simulink model "Tractor_BURGERS_etrailer_v2_1_backup070824"  (R2023a)
settings: Solver=VariableStepAuto  StartTime=0.0  StopTime=tmax  FixedStep=dt  RelTol=1e-3  EnableMultiTasking=on
PreLoadFcn:
  | init_vehicle
  | SIMSCAPE_BE_driveline_etrailer_parameters
StartFcn:
  | tic
StopFcn:
  | toc
  | sim_stop_function
  | Etrailer_Simscape_MBM_plotting
undefined symbols (not defined in the file): brake_input, chassis_length, Diesel_density, Eff, end_val, energyCapacity, etrailer_ON, final_x, final_y, Floor, front_overhang, G_motor, initialSOC, InputSwitch, L_0f, LD, mass_trailer, massload, MaxTrqOut, pose_t0, RPM, sp_t, Std_Regen_Trq, steer_input, steer_path, steer_ratio, steer_sens, throttle_input, tire_param_drive, tire_param_steer, tire_param_trailer, tire_width, Torq, v_0, Voc, Vx, Vx_input, wheelbase, X, Y, Z
libraries: sm_lib x367, nesl_utility x282, fl_lib x20, sdl_lib x2, ee_lib x2, robotalgslib x1, simulink_extras x1, batteryecm_lib x1, BatteryEstimators x1, CommercialVehicleLibrary2G x1
(part 1 of 12)
settings Model: SimulationMode=accelerator  Creator=ajayk  LastModifiedBy=utqct
settings SolverCC: AlgebraicLoopSolver=TrustRegion  EnableFixedStepZeroCrossing=on
settings DataIOCC: SaveOutput=off  ReturnWorkspaceOutputs=off  OutputTimes=[0:dt:tmax]
settings OptimizationCC: ReuseModelBlockBuffer=off
settings DebuggingCC: UnconnectedInputMsg=warning  UnconnectedOutputMsg=warning  UnconnectedLineMsg=warning
settings ModelReferenceCC: EnableRefExpFcnMdlSchedulingChecks=on  ModelReferenceMinAlgLoopOccurrences=on  PropagateSignalLabelsOutOfModel=off
settings RTWCC: DLArmComputeVersion=19.05
settings ExplorerConfigSet: InternalSimMechanicsExplorerSettings="<ExplorerConfiguration><canonicalview>default</canonicalview><AnimationSetting><BasePlaybackSpeed>1.0</BasePlaybackSpeed><PlaybackSpeedFactor>1.0</PlaybackSpeedFactor></AnimationSetting><TilePanel><TileInfo><Tiles Columns=\"2\" Count=\"4\" Rows=\"2\"><Column Weight=\"0.4998\"/><Column Weight=\"0.5002\"/><Row Weight=\"0.4996\"/><Row Weight=\"0.5004\"/><Tile Height=\"1\" Width=\"1\" X=\"0\" Y=\"0\"/><Tile Height=\"1\" Width=\"1\" X=\"0\" Y=\"1\"/><Tile Height=\"1\" Width=\"1\" X=\"1\" Y=\"0\"/><Tile Height=\"1\" Width=\"1\" X=\"1\" Y=\"1\"/></Tiles></TileInfo><SceneInfo><SceneViewer><BGColor><R>0.60000002384185791</R><G>0.60000002384185791</G><B>0.60000002384185791</B></BGColor><Camera><DoPerspective>on</DoPerspective><Position><X>56.8665384884204599</X><Y>-2.84719026045768331</Y><Z>9.20116537828617886</Z></Position><Center><X>69.9846617418789947</X><Y>-1.38429990319231133</Y><Z>2.43451606644341334</Z></Center><Up><X>-0.00100869260922395497</X><Y>0.00395248065176302329</Y><Z>0.999991680183349052</Z></Up><ViewLimDist>1</ViewLimDist><YLim>0.466307658154998583</YLim><XLim>0.60592484783857492</XLim></Camera></SceneViewer><SceneViewer><BGColor><R>0.60000002384185791</R><G>0.60000002384185791</G><B>0.60000002384185791</B></BGColor><Camera><DoPerspective>on</DoPerspective><Position><X>86.2648268522901986</X><Y>3.34890919485351812</Y><Z>3.89652789575607894</Z></Position><Center><X>81.5756793363630948</X><Y>-0.120969500296235044</Y><Z>0.901225337612659883</Z></Center><Up><X>0</X><Y>0</Y><Z>1</Z></Up><ViewLimDist>1</ViewLimDist><YLim>0.466307658154998583</YLim><XLim>0.604142715933167262</XLim></Camera></SceneViewer><SceneViewer><BGColor><R>0.60000002384185791</R><G>0.60000002384185791</G><B>0.60000002384185791</B></BGColor><Camera><DoPerspective>on</DoPerspective><Position><X>71.6158396445090943</X><Y>-1.05753967013537276</Y><Z>6.89492449835947241</Z></Position><Center><X>72.6112995913186694</X><Y>-0.962360365612823565</Y><Z>6.89555242231523646</Z></Center><Up><X>0</X><Y>0</Y><Z>1</Z></Up><ViewLimDist>1</ViewLimDist><YLim>0.466307658154998583</YLim><XLim>0.60592484783857492</XLim></Camera></SceneViewer><SceneViewer><BGColor><R>0.60000002384185791</R><G>0.60000002384185791</G><B>0.60000002384185791</B></BGColor><Camera><DoPerspective>off</DoPerspective><Position><X>498.971788791965594</X><Y>-612.498396997454847</Y><Z>371.186265282447721</Z></Position><Center><X>112.172938697542349</X><Y>-97.6356498049658938</Y><Z>57.1176303039157318</Z></Center><Up><X>-0.210251690555339377</X><Y>0.389136805237511041</Y><Z>0.896864969450900995</Z></Up><ViewLimDist>1</ViewLimDist><YLim>20.7962277663018469</YLim><XLim>26.943348032517541</XLim></Camera></SceneViewer></SceneInfo></TilePanel><MechEditorPanel><Cameras><Camera><Id>Camera1</Id><Value><Name>Side Cabin</Name><NativeCamera><PositionTrackingFeature>Tractor_semitrailer.Tractor.Cameras.Side_Camera_Sphere.R</PositionTrackingFeature><CenterTrackingFeature>Tractor_semitrailer.Tractor.World.Chassis</CenterTrackingFeature><UpVectorTrackingFeature>Tractor_semitrailer.Tractor.World.x6_DOF_Joint.B</UpVectorTrackingFeature><CenterTrackingOrigin>on</CenterTrackingOrigin><UpVectorTrackingDirection>+Z</UpVectorTrackingDirection></NativeCamera></Value></Camera><Camera><Id>Camera2</Id><Value><Name>Top  Cabin</Name><NativeCamera><PositionTrackingFeature>Tractor_semitrailer.Tractor.Cameras.Front_Camera_Transform.F</PositionTrackingFeature><CenterTrackingFeature>Tractor_semitrailer.Tractor.Cabin.Brick_Solid.R</CenterTrackingFeature><UpVectorTrackingFeature>Tractor_semitrailer.Tractor.World.x6_DOF_Joint.B</UpVectorTrackingFeature><CenterTrackingOrigin>off</CenterTrackingOrigin><CenterTrackingDirection>+X</CenterTrackingDirection><UpVectorTrackingDirection>+Z</UpVectorTrackingDirection></NativeCamera></Value></Camera><Camera><Id>Camera3</Id><Value><Name>Trailer Top</Name><NativeCamera><PositionTrackingFeature>Tractor_semitrailer.Semitrailer.Cameras.Trailer_Camera_Position.F</PositionTrackingFeature><CenterTrackingFeature>Tractor_semitrailer.Semitrailer.Trailer_load_rear.Load.R</CenterTrackingFeature><UpVectorTrackingFeature>Tractor_semitrailer.Semitrailer.x5th_Wheel</UpVectorTrackingFeature><CenterTrackingOrigin>on</CenterTrackingOrigin><UpVectorTrackingDirection>+Z</UpVectorTrackingDirection></NativeCamera></Value></Camera></Cameras><GfxPanelCameraMap><MapElement CameraMLId=\"Camera3\" GfxPanelIndex=\"0\"/><MapElement CameraMLId=\"Camera1\" GfxPanelIndex=\"1\"/><MapElement CameraMLId=\"Camera2\" GfxPanelIndex=\"2\"/></GfxPanelCameraMap><VideoCreator><PlaybackSpeedRatio>1.0</PlaybackSpeedRatio><FrameRate>30</FrameRate><VideoFormat>Motion JPEG AVI</VideoFormat><FrameSize>auto</FrameSize></VideoCreator></MechEditorPanel></ExplorerConfiguration>"

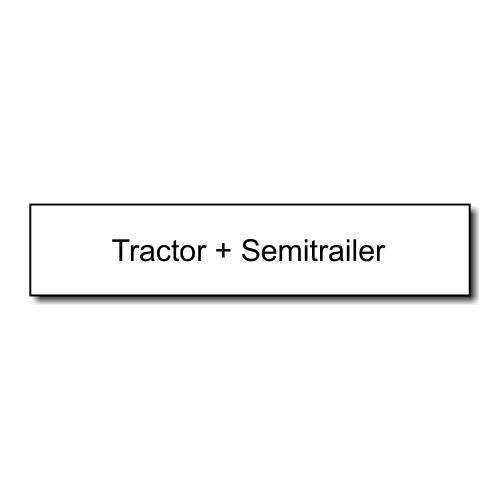
[thumbnail: Simulink's stored preview of the top-level diagram]
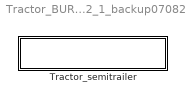
== system Tractor_BURGERS_etrailer_v2_1_backup070824 ==
  "Tractor_semitrailer " : Subsystem
      mask Display: disp('Tractor + Semitrailer')

== system Tractor_BURGERS_etrailer_v2_1_backup070824/Tractor_semitrailer  ==
  Bus Selector : BusSelector  OutputSignals=chassis.Vx,steeraxle.pos.X,steeraxle.pos.Y,world.yaw
  Clock : Clock
  Driver : Subsystem
      settings: LibrarySourceBlock=CommercialVehicleLibrary2G/Assemblies/Driver
  Gain1 : Gain  Gain=100
  Gain2 : Gain  Gain=100
  Kraker etrailer : Subsystem  mask(semitrailer (3 non-steered axles)){xref=-3.06, xaxle2=wheelbase, lchassis=chassis_length, x5th=front_overhang, mass_empty=mass_trailer, mass_load=massload, rho=350, Fzstat=7000*9.81, lbdouble=0, psi_semitrailer=pose_t0(4)}
      mask prompts: xref "Global X-coordinate 5th wheel [m]"; xaxle2 "Distance 5th wheel to second semitrailer axle [m]"; lchassis "Semitrailer chassis length [m]"; x5th "Distance front trailer to 5th wheel [m]"; mass_empty "Mass of empty semitrailer [kg]"; mass_load "Mass of load [kg]"; rho "Density of load [kg/m3]"; Fzstat "Initial vertical axle load [N]"; lbdouble "B-double load length reduction (rear side) [m]"; psi_semitrailer "Articulation angle (t=0) [rad]"
      mask init:
      | %Semitrailer chassis
      | xcg1  = xref+x5th-0.25*lchassis;            % [m], Center of the first semitrailer chassis wrt global axis system
      | xcg2  = xref+x5th-0.75*lchassis;            % [m], Center of the second semitrailer chassis wrt global axis system
      | xrev1 = xref+x5th-0.5*lchassis;             % [m], Position of torsional spring wrt global axis system
      | 
      | l=0.5*lchassis;
      | w=1.5;
      | h=0.3;
      | chassis_mass= (mass_empty-3*650)/2;         % [kg] 
      | chassis_Ixx = chassis_mass*(w*w+h*h)/12;    % [kgm2]
      | chassis_Iyy = chassis_mass*(l*l+h*h)/12;    % [kgm2]
      | chassis_Izz = chassis_mass*(l*l+w*w)/12;    % [kgm2]
      | 
      | %Loading
      | l_load1 = 0.5*lchassis;
      | l_load2 = 0.5*lchassis-lbdouble;
      | xload1  = xref+x5th-0.5*l_load1;             % [m], Global X-coordinate center of load1
      | xload2  = xref+x5th-0.5*l_load2-l_load1;     % [m], Global X-coordinate center of load2
      | 
      | mass_load1 = l_load1/(l_load1+l_load2)*mass_load;
      | mass_load2 = l_load2/(l_load1+l_load2)*mass_load;
      settings: LibrarySourceBlock=CommercialVehicleLibrary2G/Trailers/Semitrailer
  To Workspace : ToWorkspace  VariableName=p_time  SampleTime=sp_t
  To Workspace21 : ToWorkspace  VariableName=p_inputs_delta  SampleTime=sp_t
  To Workspace22 : ToWorkspace  VariableName=p_inputs_throttle  SampleTime=sp_t
  To Workspace23 : ToWorkspace  VariableName=p_inputs_brake  SampleTime=sp_t
  To_workspace_semitrailer : Subsystem
      settings: LibrarySourceBlock=CommercialVehicleLibrary2G/Utilities/To_workspace_semitrailer
      mask Display: disp('Workspace - Semitrailer')
  To_workspace_tractor : Subsystem
      mask Display: disp('Workspace - Tractor')
  Tractor : Subsystem  mask{xref=0, xrear=-3.80, Fzstat1=7500*9.81, Fzstat2=11500*9.81, Xt0=pose_t0(1), Yt0=pose_t0(2), Psit0=pose_t0(3)}
      mask prompts: xref "Global X-coordinate front axle [m]"; xrear "X-coordinate rear axle (relative to front) [m]"; Fzstat1 "Steer Axle Initial Vertical Axle Load [N]"; Fzstat2 "Drive Axle Initial Vertical Axle Load [N]"; Xt0 "Global X-position front axle tractor [m]"; Yt0 "Global Y-position front axle tractor [m]"; Psit0 "Heading angle tractor [rad]"
      mask init:
      | % Torsional joint 
      | x_torsion = xref-1.3;   % [m],X-coordinate torsional joint wrt reference point
      | 
      | % Front part of vehicle chassis
      | l1=2.6;
      | w1=1.0;
      | h1=0.3;
      | xcg_front  = xref;   % [m],X-coordinate C.G. wrt reference point
      | front_mass = 1349;   % [kg]
      | front_Ixx  = front_mass*(w1*w1+h1*h1)/12;    % [kgm2]
      | front_Iyy  = front_mass*(l1*l1+h1*h1)/12;    % [kgm2]
      | front_Izz  = front_mass*(l1*l1+w1*w1)/12;    % [kgm2]
      | 
      | % Rear part of vehicle chassis
      | l2=3.3;
      | w2=1.0;
      | h2=0.3;
      | xcg_rear  = xref-1.3 - 0.5*l2;          % [m], global X-coordinate CG 
      | rear_mass = 400;                       % [kg] 
      | rear_Ixx  = rear_mass*(w2*w2+h2*h2)/12;    % [kgm2]
      | rear_Iyy  = rear_mass*(l2*l2+h2*h2)/12;    % [kgm2]
      | rear_Izz  = rear_mass*(l2*l2+w2*w2)/12;    % [kgm2]
      settings: LibrarySourceBlock=CommercialVehicleLibrary2G/Vehicles/Tractor
      mask DialogControl IniPos Prompt: Initial vehicle position (At t=0 sec.)
  wires:
  Clock/1 -> To Workspace/1, Driver/1(time)
  Tractor/1(Signals) -> Bus Selector/1, To_workspace_tractor/1(In1)
  Kraker etrailer/1(Signals) -> To_workspace_semitrailer/1(In1)
  Bus Selector/4 -> Driver/5(Yaw)  "<yaw>"
  Bus Selector/1 -> [Vx], Driver/2(Vx)  "<Vx>"
  Bus Selector/2 -> Driver/3("FrontAxlePosX ")  "<X>"
  Bus Selector/3 -> Driver/4(FrontAxlePosY)  "<Y>"
  Driver/2(Throttle) -> Gain1/1, Tractor/2(Throttle), [throttle]
  Driver/3(Brake) -> [brake], Tractor/3(Brake), Gain2/1
  Driver/1(Steering) -> To Workspace21/1, Tractor/1(Steering)
  [Vx] -> Kraker etrailer/1(Vx)
  Gain2/1 -> To Workspace23/1
  Gain1/1 -> To Workspace22/1
  Kraker etrailer/2(DriveTrqs_etrailer) -> Tractor/4(DriveTrqs_etrailer)
  Tractor/2(Mb_trailer) -> Kraker etrailer/2(Mb_trailer)
  [throttle] -> Kraker etrailer/3(throttle)
  [brake] -> Kraker etrailer/4(brake)
  [Vx] -> Tractor/5(Vx)
  connections:
  Kraker etrailer/LConn1 -- Tractor/RConn1
  Kraker etrailer/LConn2 -- Tractor/RConn2

== system Tractor_BURGERS_etrailer_v2_1_backup070824/Tractor_semitrailer /Driver ==
  time : Inport
  Vx : Inport  Port=2
  "FrontAxlePosX " : Inport  Port=3
  FrontAxlePosY : Inport  Port=4
  Yaw : Inport  Port=5
  Abs : Abs  SaturateOnIntegerOverflow=off
  Constant : Constant  Value=0
  Constant1 : Constant  Value=max(throttle_input(2,:))
  Constant2 : Constant  Value=max(abs(steer_path(:,2)))
  Constant3 : Constant  Value=steer_path
  Control : Subsystem
  CruiseControl : Subsystem
  Saturation : Saturate  UpperLimit=0  LowerLimit=-1
  Saturation1 : Saturate  UpperLimit=1  LowerLimit=0
  Subsystem : Subsystem
  Switch : Switch  Threshold=0.0001  SaturateOnIntegerOverflow=off  InputSameDT=off
  Switch1 : Switch  Threshold=0.0001  SaturateOnIntegerOverflow=off  InputSameDT=off
  Switch2 : Switch  Threshold=0.0001  SaturateOnIntegerOverflow=off  InputSameDT=off
  Terminator : Terminator
  Vx_input : Lookup  InputValues=Vx_input(1,:)  Table=Vx_input(2,:)  SaturateOnIntegerOverflow=off
  brake_input : Lookup  InputValues=brake_input(1,:)  Table=brake_input(2,:)  SaturateOnIntegerOverflow=off
  steer_input : Lookup  InputValues=steer_input(1,:)  Table=steer_input(2,:)  SaturateOnIntegerOverflow=off
  throttle_input : Lookup  InputValues=throttle_input(1,:)  Table=throttle_input(2,:)  SaturateOnIntegerOverflow=off
  Steering : Outport  VectorParamsAs1DForOutWhenUnconnected=off
  Throttle : Outport  Port=2  VectorParamsAs1DForOutWhenUnconnected=off
  Brake : Outport  Port=3  VectorParamsAs1DForOutWhenUnconnected=off
  wires:
  brake_input/1 -> Switch/2
  Constant/1 -> Switch/1
  time/1 -> brake_input/1, Vx_input/1, throttle_input/1, steer_input/1
  Switch/1 -> Saturation1/1
  Constant1/1 -> Switch1/2
  Switch1/1 -> Saturation/1, Switch/3
  CruiseControl/1(throttle) -> Switch1/3
  throttle_input/1 -> Switch1/1
  Vx/1 -> CruiseControl/2(Vx,actual)
  steer_input/1 -> Switch2/3
  Constant2/1 -> Switch2/2
  Constant3/1 -> Control/1(path)
  Control/1(delta in rad) -> Switch2/1
  "FrontAxlePosX "/1 -> Control/2(truck_x)
  FrontAxlePosY/1 -> Control/3(truck_y)
  Yaw/1 -> Control/4(truck_yaw)
  Switch2/1 -> Steering/1  "rad"
  Subsystem/1(DriveCycleInput) -> CruiseControl/1(Vx,ref)
  Saturation/1 -> Abs/1
  Abs/1 -> Brake/1
  Vx_input/1 -> Terminator/1
  Saturation1/1 -> Throttle/1

== system Tractor_BURGERS_etrailer_v2_1_backup070824/Tractor_semitrailer /Kraker etrailer ==
  Vx : Inport
  Mb_trailer : Inport  Port=2
  throttle : Inport  Port=3
  brake : Inport  Port=4
  5th Wheel Joint : Subsystem
      mask Display: disp('5th Wheel Joint');
  Bus Creator : BusCreator  Inputs=8
  Cameras : Subsystem
      settings: PortSchema="{\"entries\":[{\"content\":{\"sides\":[{\"content\":{\"connectorIds\":[]},\"type\":\"ConnectorPlacement.EquallySpacedRectSide\",\"uuid\":\"323b7ff6-2456-4e2e-a0c0-1caaddbc2339\"},{\"content\":{\"connectorIds\":[],\"side\":\"RIGHT\"},\"type\":\"ConnectorPlacement.EquallySpacedRectSide\",\"uuid\":\"1f5e267e-0c09-46b4-9116-e9355f2454eb\"},{\"content\":{\"connectorIds\":[],\"side\":\"TOP\"},\"type\":\"ConnectorPlacement.EquallySpacedRectSide\",\"uuid\":\"bb2ab4c9-7fc2-4cfd-82e7-e1d9a115e820\"},{\"content\":{\"connectorIds\":[\"RConn1\"],\"side\":\"BOTTOM\"},\"type\":\"ConnectorPlacement.EquallySpacedRectSide\",\"uuid\":\"8ef0eb7c-e2ec-48d5-a68d-8a9419d00a1f\"}]},\"type\":\"ConnectorPlacement.EquallySpacedConnector\",\"uuid\":\"9bf912c0-916c-4d24-bea5-037dc0fe3be9\"}],\"packageUris\":[\"http://schema.mathworks.com/mf0/Connector/R2020b\"],\"version\":\"1.0\"}"
  Electric Powertrain : Subsystem
      settings: PortSchema="{\"entries\":[{\"content\":{\"sides\":[{\"content\":{\"connectorIds\":[\"In1\"]},\"type\":\"ConnectorPlacement.EquallySpacedRectSide\",\"uuid\":\"157e9ca7-4557-4784-80e8-a2717cc996a6\"},{\"content\":{\"connectorIds\":[\"RConn1\",\"RConn2\",\"Out1\"],\"side\":\"RIGHT\"},\"type\":\"ConnectorPlacement.EquallySpacedRectSide\",\"uuid\":\"8309c863-b11c-42d5-89d5-fce448da9e7d\"},{\"content\":{\"side\":\"TOP\"},\"type\":\"ConnectorPlacement.EquallySpacedRectSide\",\"uuid\":\"8590e6de-18e9-4364-8df4-b601f0af8074\"}]},\"type\":\"ConnectorPlacement.EquallySpacedConnector\",\"uuid\":\"5fa93450-c38b-434f-93e4-f6394569ac9a\"}],\"packageUris\":[\"http://schema.mathworks.com/mf0/Connector/R2020b\"],\"version\":\"1.0\"}"
  Etrailer-Controller : Subsystem
  Subsystem : Subsystem
  To origin (For further articulation) : sm_lib/Frames and Transforms/Rigid Transform  Commented=on  TranslationMethod=Cartesian  TranslationStandardOffset=0  TranslationStandardOffsetUnits=m  TranslationStandardAxis=+Z  TranslationCartesianOffset=[-xcg2 0 -1.2]  TranslationCartesianOffsetUnits=m  TranslationROffset=0  TranslationROffsetUnits=m  TranslationZOffset=0  TranslationZOffsetUnits=m  TranslationThetaOffset=0  TranslationThetaOffsetUnits=deg  RotationMethod=None  RotationAngleUnits=deg  RotationStandardAxis=+Z  RotationAngle=0.0  RotationArbitraryAxis=[0 0 1]  FollAlignAxisA=+X  BaseAlignAxisA=+Y  FollAlignAxisB=+Y  BaseAlignAxisB=+Z  RotationSequenceAxes=FollowerAxes  RotationSequence=XYX  RotationSequenceAngles=[0 0 0]  RotationSequenceAnglesUnits=deg  RotationMatrix=[1 0 0; 0 1 0; 0 0 1]  Quaternion=[1 0 0 0]
  Trailer axle 1 : Subsystem  mask(Axle with single tyres){xpos=xref-xaxle2+1.40, tire_param=tire_param_trailer, Vx=Vx, Fzstat=Fzstat}
      mask prompts: xpos "global X-coordinate wheelcentre [m]"; tire_param "Tire parameters"; Vx "initial velocity Vx [m/s]"; Fzstat "initial vertical axle load [N]"
      mask init:
      | Rtyre     = 0.546;
      | Cztyre    = 1.35e+006;
      | tyre_mass= tire_param.INERTIA.MASS;
      | 
      | zpos   =Rtyre - 0.5*Fzstat/Cztyre;
      | 
      | % dimensions
      | tw =2.0;  % [m], track_width
      | yd =1.0;  % [m], Y-distance bewteen dampers
      | ys =1.0;  % [m], Y-distance bewteen springs 
      | zrc=0.2;  % [m], height of roll centre wrt axle 
      |    
      | % damping/stiffness
      | Kspring = 394000;  % [N/m], spring stiffness (two per axle!)
      | Bdamper =  20000;  % [Ns/m] damper constant (two per axle!)
      | Kroll   =1516000;  % [Nm/rad] roll stiffness 
      |    
      | % mass/inertia
      | axle_mass = 400;  % [kg]
      | axle_Ixx  = 200; % [kgm2]
      | axle_Iyy  =  10;   % [kgm2]
      | axle_Izz  = 200; % [kgm2]
      |    
      | rim_mass= 55; % [kg]
      | rim_Ixx =  4; % [kgm2]
      | rim_Iyy =  6; % [kgm2] (including rotational inertia brake disk)
      | 
      | %WHeel mass 
      | wheelbody_mass = rim_mass + tire_param.INERTIA.MASS;
      | wheelbody_Ixx  = rim_Ixx  + tire_param.INERTIA.IXX;
      | wheelbody_Iyy  = rim_Iyy  + tire_param.INERTIA.IYY;
      | Imat = [wheelbody_Ixx 0 0; 0 wheelbody_Iyy 0; 0 0 wheelbody_Ixx];
      | sideR=-1;
      | sideL=1;
      | 
      | ld = 0.3;                     % loaded spring/damper length
      | ls = ld + 0.5*(Fzstat - 9.81*(axle_mass + 2*tyre_mass + 2*rim_mass))/Kspring;  % spring unloaded length
  Trailer axle 2 : Subsystem  mask(Axle with single tyres){xpos=xref-xaxle2, tire_param=tire_param_trailer, Vx=Vx, Fzstat=Fzstat}
      mask prompts: xpos "global X-coordinate wheelcentre [m]"; tire_param "tyre parameters"; Vx "initial velocity Vx [m/s]"; Fzstat "initial vertical axle load [N]"
      mask init: same as Tractor_BURGERS_etrailer_v2_1_backup070824/Tractor_semitrailer /Kraker etrailer/Trailer axle 1
      settings: LibrarySourceBlock=CommercialVehicleLibrary2G/Assemblies/Trailer axle
  Trailer axle 3 : Subsystem  mask(Axle with single tyres){xpos=xref-xaxle2-1.40, tire_param=tire_param_trailer, Vx=Vx, Fzstat=Fzstat}
      mask prompts: xpos "global X-coordinate wheelcentre [m]"; tire_param "Tire parameters"; Vx "initial velocity Vx [m/s]"; Fzstat "initial vertical axle load [N]"
      mask init: same as Tractor_BURGERS_etrailer_v2_1_backup070824/Tractor_semitrailer /Kraker etrailer/Trailer axle 1
      settings: LibrarySourceBlock=CommercialVehicleLibrary2G/Assemblies/Trailer axle
  Trailer load front : Subsystem  mask{xload=xload1, zload=1.3, mass_load=mass_load1, l_load=l_load1, w=2.5, rho=rho}
      mask prompts: xload "Global X-coordinate Center of Load [m]"; zload "Global Z-coordinate Application of Load [m]"; mass_load "mass [kg]"; l_load "length [m]"; w "width [m]"; rho "density [kg/m3]"
      mask init:
      | h=(mass_load)/(rho*w*(l_load));
      | zcg=0.5*h;
      | Ixx=(mass_load)*(w*w+h*h)/12;
      | Iyy=(mass_load)*((l_load)*(l_load)+h*h)/12;
      | Izz=(mass_load)*((l_load)*(l_load)+w*w)/12;
      mask Display: disp('Trailer front load ')
  Trailer load rear : Subsystem  mask{xload=xload2, zload=1.3, mass_load=mass_load2, l_load=l_load2, w=2.5, rho=rho}
      mask prompts: xload "Global X-coordinate Center of Load [m]"; zload "Global Z-coordinate Application of Load [m]"; mass_load "mass [kg]"; l_load "length [m]"; w "width [m]"; rho "density [kg/m3]"
      mask init:
      | h=(mass_load)/(rho*w*(l_load));
      | zcg=0.5*h;
      | Ixx=(mass_load)*(w*w+h*h)/12;
      | Iyy=(mass_load)*((l_load)*(l_load)+h*h)/12;
      | Izz=(mass_load)*((l_load)*(l_load)+w*w)/12;
      mask Display: disp('Trailer rear load ')
  Trailer_front : sm_lib/Body Elements/Brick Solid  GraphicAmbientColor=[0.15 0.15 0.15 1.0]  BasedOnType=Density  BrickDimensions=[l w h]  BrickDimensionsUnits=m  CenterOfMass=[0 0 0]  CenterOfMassUnits=m  GraphicDiffuseColor=[0.4 0.4 0.4]  Density=1000  DensityUnits=kg/m^3  DoExposeReferenceFrame=on  GraphicEmissiveColor=[0.0 0.0 0.0 1.0]  ExportEntireGeometry=off  SerializedFrames=<Frames><Frame><Id>Frame1</Id><Value><Name>F1</Name><Origin><Source>ReferenceFrame</Source><FeatureName></FeatureName></Origin><PrimaryAxis><DefinedDirection>+Z</DefinedDirection><Source>ReferenceFrame</Source><SourceDirection>+Z</SourceDirection><FeatureName></FeatureName></PrimaryAxis><SecondaryAxis><DefinedDirection>+X</DefinedDirection><Source>ReferenceFrame</Source><SourceDirection>+X</SourceDirection><FeatureName></FeatureName></SecondaryAxis></Value></Frame></Frames>  MarkerShape=Sphere  MarkerSize=10  GraphicType=FromGeometry  InertiaType=Custom  Mass=chassis_mass  MassUnits=kg  MomentsOfInertia=[chassis_Ixx chassis_Iyy chassis_Izz]  MomentsOfInertiaUnits=kg*m^2  GraphicOpacity=1  ProductsOfInertia=[0 0 0]  ProductsOfInertiaUnits=kg*m^2  GraphicShininess=75  GraphicSpecularColor=[0.5 0.5 0.5 1.0]  GraphicVisPropType=SimpleVisualProperties
  Trailer_rear : sm_lib/Body Elements/Brick Solid  GraphicAmbientColor=[0.15 0.15 0.15 1.0]  BasedOnType=Density  BrickDimensions=[l w h]  BrickDimensionsUnits=m  CenterOfMass=[0 0 0]  CenterOfMassUnits=m  GraphicDiffuseColor=[0.9 0.9 0.9]  Density=1000  DensityUnits=kg/m^3  DoExposeReferenceFrame=on  GraphicEmissiveColor=[0.0 0.0 0.0 1.0]  ExportEntireGeometry=off  SerializedFrames=<Frames><Frame><Id>Frame1</Id><Value><Name>F1</Name><Origin><Source>ReferenceFrame</Source><FeatureName></FeatureName></Origin><PrimaryAxis><DefinedDirection>+Z</DefinedDirection><Source>ReferenceFrame</Source><SourceDirection>+Z</SourceDirection><FeatureName></FeatureName></PrimaryAxis><SecondaryAxis><DefinedDirection>+X</DefinedDirection><Source>ReferenceFrame</Source><SourceDirection>+X</SourceDirection><FeatureName></FeatureName></SecondaryAxis></Value></Frame></Frames>  MarkerShape=Sphere  MarkerSize=10  GraphicType=FromGeometry  InertiaType=Custom  Mass=chassis_mass  MassUnits=kg  MomentsOfInertia=[chassis_Ixx chassis_Iyy chassis_Izz]  MomentsOfInertiaUnits=kg*m^2  GraphicOpacity=0.8  ProductsOfInertia=[0 0 0]  ProductsOfInertiaUnits=kg*m^2  GraphicShininess=75  GraphicSpecularColor=[0.5 0.5 0.5 1.0]  GraphicVisPropType=SimpleVisualProperties
  Trailer_torsion : Subsystem
      settings: PortSchema="{\"entries\":[{\"content\":{\"sides\":[{\"content\":{\"connectorIds\":[\"LConn1\"]},\"type\":\"ConnectorPlacement.EquallySpacedRectSide\",\"uuid\":\"b43c74bd-af15-4ffb-863b-6a132848d787\"},{\"content\":{\"connectorIds\":[\"RConn1\"],\"side\":\"RIGHT\"},\"type\":\"ConnectorPlacement.EquallySpacedRectSide\",\"uuid\":\"8ef5ae9f-2f99-4b38-816f-c2fb0756fe1b\"},{\"content\":{\"connectorIds\":[\"Out1\",\"Out2\"],\"side\":\"TOP\"},\"type\":\"ConnectorPlacement.EquallySpacedRectSide\",\"uuid\":\"649c363b-e78d-45fa-ac8c-bda3eda724e3\"},{\"content\":{\"connectorIds\":[],\"side\":\"BOTTOM\"},\"type\":\"ConnectorPlacement.EquallySpacedRectSide\",\"uuid\":\"5c9a8245-60cb-4b5f-86c5-abbc61b03337\"}]},\"type\":\"ConnectorPlacement.EquallySpacedConnector\",\"uuid\":\"06fb9ebd-5177-4420-93bb-82569f181fb4\"}],\"packageUris\":[\"http://schema.mathworks.com/mf0/Connector/R2020b\"],\"version\":\"1.0\"}"
      mask Display: disp('Torsion');
  5th Wheel : PMIOPort  Tag=PMCPort  Side=Left
  Ground : PMIOPort  Port=2  Side=Left
  Signals : Outport
  DriveTrqs_etrailer : Outport  Port=2
  wires:
  [semitrailerload2] -> Bus Creator/5  "load2"
  [semitrailerload1] -> Bus Creator/4  "load1"
  [axle3] -> Bus Creator/3  "axle3"
  [axle2] -> Bus Creator/2  "axle2"
  [axle1] -> Bus Creator/1  "axle1"
  Trailer axle 3/1(signals) -> [axle3]
  Trailer axle 2/1(signals) -> [axle2]
  Trailer axle 1/1(signals) -> [axle1]
  Bus Creator/1 -> Signals/1
  [torsion] -> Bus Creator/6  "torsion"
  Trailer load rear/1(signals) -> [semitrailerload2]
  Trailer load front/1(signals) -> [semitrailerload1]
  Trailer_torsion/1(Signals) -> [torsion]
  [kingpin] -> Bus Creator/7  "kingpin"
  5th Wheel Joint/1(signals) -> [kingpin]  "kingpin forces"
  Trailer_torsion/2(signals) -> [Rotation]  "Rotation"
  [Rotation] -> Bus Creator/8  "Rotation"
  Subsystem/1(DriveCycleInput) -> Etrailer-Controller/1(RefVehSpeed)
  Etrailer-Controller/2(MotorCmdTrq) -> Electric Powertrain/1(MotCmdTrq)
  Etrailer-Controller/1(Mb) -> Trailer axle 1/1(Mb), Trailer axle 3/1(Mb), Trailer axle 2/1(Mb)
  Vx/1 -> Etrailer-Controller/2(Vx)
  Trailer axle 2/2(DriveTrqs_etrailer) -> DriveTrqs_etrailer/1
  brake/1 -> Etrailer-Controller/4(brake)
  throttle/1 -> Etrailer-Controller/3(throttle)
  Mb_trailer/1 -> Etrailer-Controller/5(Mb_trailer)
  Electric Powertrain/1(SOC) -> Etrailer-Controller/6(SOC)
  connections:
  Trailer_rear/LConn1 -- Trailer axle 1/LConn1 -- Trailer axle 2/LConn1 -- Trailer axle 3/LConn1 -- Trailer load rear/LConn1 -- To origin (For further articulation)/LConn1
  5th Wheel Joint/RConn1 -- Trailer_front/RConn1
  Trailer_torsion/LConn1 -- Cameras/RConn1 -- Trailer load front/LConn1 -- Trailer_front/LConn1
  5th Wheel Joint/LConn1 -- 5th Wheel/RConn1
  Trailer_rear/RConn1 -- Trailer_torsion/RConn1
  Trailer axle 2/LConn2 -- Trailer axle 3/LConn2 -- Ground/RConn1 -- Trailer axle 1/LConn2
  Electric Powertrain/RConn1 -- Trailer axle 2/LConn3
  Electric Powertrain/RConn2 -- Trailer axle 2/LConn4

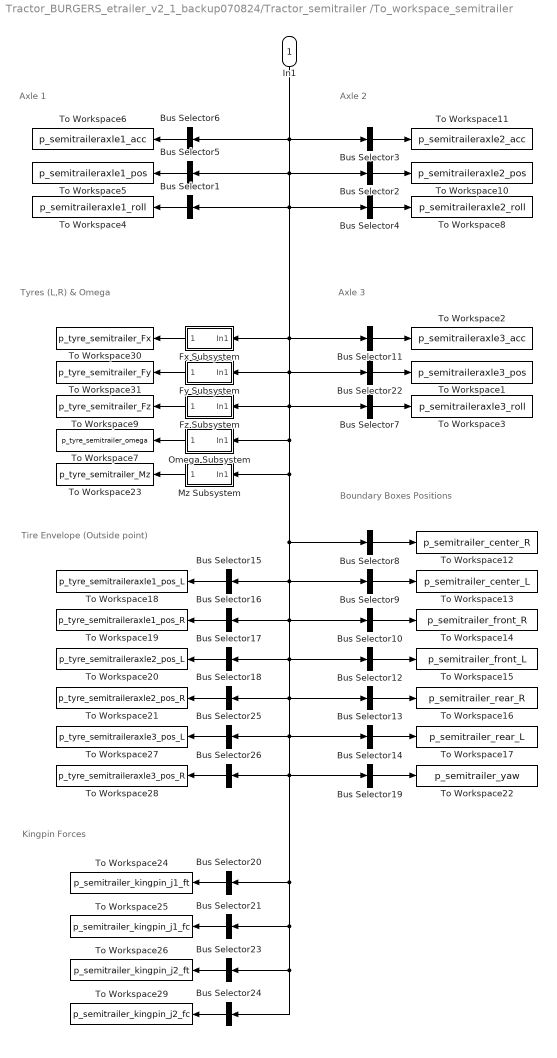
== system Tractor_BURGERS_etrailer_v2_1_backup070824/Tractor_semitrailer /To_workspace_semitrailer ==
  note: Kingpin Forces
  note: Tire Envelope (Outside point)
  note: Boundary Boxes Positions
  note: Tyres (L,R) & Omega
  note: Axle 3
  note: Axle 2
  note: Axle 1
  In1 : Inport
  Bus Selector1 : BusSelector  OutputSignals=axle1.Axle_roll  OutputAsBus=on
  Bus Selector10 : BusSelector  OutputSignals=load1.pos_FR  OutputAsBus=on
  Bus Selector11 : BusSelector  OutputSignals=axle3.Axle_acc  OutputAsBus=on
  Bus Selector12 : BusSelector  OutputSignals=load1.pos_FL  OutputAsBus=on
  Bus Selector13 : BusSelector  OutputSignals=load2.pos_RR  OutputAsBus=on
  Bus Selector14 : BusSelector  OutputSignals=load2.pos_RL  OutputAsBus=on
  Bus Selector15 : BusSelector  OutputSignals=axle1.T_L_pos  OutputAsBus=on
  Bus Selector16 : BusSelector  OutputSignals=axle1.T_R_pos  OutputAsBus=on
  Bus Selector17 : BusSelector  OutputSignals=axle2.Tire_L_pos  OutputAsBus=on
  Bus Selector18 : BusSelector  OutputSignals=axle2.Tire_R_pos  OutputAsBus=on
  Bus Selector19 : BusSelector  OutputSignals=Rotation.yaw  OutputAsBus=on
  Bus Selector2 : BusSelector  OutputSignals=axle2.Axle_pos  OutputAsBus=on
  Bus Selector20 : BusSelector  OutputSignals=kingpin.ft_joint1  OutputAsBus=on
  Bus Selector21 : BusSelector  OutputSignals=kingpin.fc_joint1  OutputAsBus=on
  Bus Selector22 : BusSelector  OutputSignals=axle3.Axle_pos  OutputAsBus=on
  Bus Selector23 : BusSelector  OutputSignals=kingpin.ft_joint2  OutputAsBus=on
  Bus Selector24 : BusSelector  OutputSignals=kingpin.fc_joint2  OutputAsBus=on
  Bus Selector25 : BusSelector  OutputSignals=axle3.Tire L Pos  OutputAsBus=on
  Bus Selector26 : BusSelector  OutputSignals=axle3.Tire R Pos  OutputAsBus=on
  Bus Selector3 : BusSelector  OutputSignals=axle2.Axle_acc  OutputAsBus=on
  Bus Selector4 : BusSelector  OutputSignals=axle2.Axle_roll  OutputAsBus=on
  Bus Selector5 : BusSelector  OutputSignals=axle1.Axle_pos  OutputAsBus=on
  Bus Selector6 : BusSelector  OutputSignals=axle1.Axle_acc  OutputAsBus=on
  Bus Selector7 : BusSelector  OutputSignals=axle3.Axle_roll  OutputAsBus=on
  Bus Selector8 : BusSelector  OutputSignals=load1.pos_CR  OutputAsBus=on
  Bus Selector9 : BusSelector  OutputSignals=load1.pos_CL  OutputAsBus=on
  Fx Subsystem : Subsystem
      mask Display: disp('Fx');
  Fy Subsystem : Subsystem
      mask Display: disp('Fy');
  Fz Subsystem : Subsystem
      mask Display: disp('Fz');
  Mz Subsystem : Subsystem
      mask Display: disp('Mz');
  Omega Subsystem : Subsystem
      mask Display: disp('Ω');
  To Workspace1 : ToWorkspace  VariableName=p_semitraileraxle3_pos  SampleTime=sp_t
  To Workspace10 : ToWorkspace  VariableName=p_semitraileraxle2_pos  SampleTime=sp_t
  To Workspace11 : ToWorkspace  VariableName=p_semitraileraxle2_acc  SampleTime=sp_t
  To Workspace12 : ToWorkspace  VariableName=p_semitrailer_center_R  SampleTime=sp_t
  To Workspace13 : ToWorkspace  VariableName=p_semitrailer_center_L  SampleTime=sp_t
  To Workspace14 : ToWorkspace  VariableName=p_semitrailer_front_R  SampleTime=sp_t
  To Workspace15 : ToWorkspace  VariableName=p_semitrailer_front_L  SampleTime=sp_t
  To Workspace16 : ToWorkspace  VariableName=p_semitrailer_rear_R  SampleTime=sp_t
  To Workspace17 : ToWorkspace  VariableName=p_semitrailer_rear_L  SampleTime=sp_t
  To Workspace18 : ToWorkspace  VariableName=p_tyre_semitraileraxle1_pos_L  SampleTime=sp_t
  To Workspace19 : ToWorkspace  VariableName=p_tyre_semitraileraxle1_pos_R  SampleTime=sp_t
  To Workspace2 : ToWorkspace  VariableName=p_semitraileraxle3_acc  SampleTime=sp_t
  To Workspace20 : ToWorkspace  VariableName=p_tyre_semitraileraxle2_pos_L  SampleTime=sp_t
  To Workspace21 : ToWorkspace  VariableName=p_tyre_semitraileraxle2_pos_R  SampleTime=sp_t
  To Workspace22 : ToWorkspace  VariableName=p_semitrailer_yaw  SampleTime=sp_t
  To Workspace23 : ToWorkspace  VariableName=p_tyre_semitrailer_Mz  SampleTime=sp_t
  To Workspace24 : ToWorkspace  VariableName=p_semitrailer_kingpin_j1_ft  SampleTime=sp_t
  To Workspace25 : ToWorkspace  VariableName=p_semitrailer_kingpin_j1_fc  SampleTime=sp_t
  To Workspace26 : ToWorkspace  VariableName=p_semitrailer_kingpin_j2_ft  SampleTime=sp_t
  To Workspace27 : ToWorkspace  VariableName=p_tyre_semitraileraxle3_pos_L  SampleTime=sp_t
  To Workspace28 : ToWorkspace  VariableName=p_tyre_semitraileraxle3_pos_R  SampleTime=sp_t
  To Workspace29 : ToWorkspace  VariableName=p_semitrailer_kingpin_j2_fc  SampleTime=sp_t
  To Workspace3 : ToWorkspace  VariableName=p_semitraileraxle3_roll  SampleTime=sp_t
  To Workspace30 : ToWorkspace  VariableName=p_tyre_semitrailer_Fx  SampleTime=sp_t
  To Workspace31 : ToWorkspace  VariableName=p_tyre_semitrailer_Fy  SampleTime=sp_t
  To Workspace4 : ToWorkspace  VariableName=p_semitraileraxle1_roll  SampleTime=-1
  To Workspace5 : ToWorkspace  VariableName=p_semitraileraxle1_pos  SampleTime=sp_t
  To Workspace6 : ToWorkspace  VariableName=p_semitraileraxle1_acc  SampleTime=sp_t
  To Workspace7 : ToWorkspace  VariableName=p_tyre_semitrailer_omega  SampleTime=sp_t
  To Workspace8 : ToWorkspace  VariableName=p_semitraileraxle2_roll  SampleTime=sp_t
  To Workspace9 : ToWorkspace  VariableName=p_tyre_semitrailer_Fz  SampleTime=sp_t
  wires:
  Bus Selector7/1 -> To Workspace3/1
  Bus Selector4/1 -> To Workspace8/1
  Bus Selector1/1 -> To Workspace4/1
  Bus Selector11/1 -> To Workspace2/1
  Bus Selector2/1 -> To Workspace10/1
  Bus Selector3/1 -> To Workspace11/1
  Fx Subsystem/1(Out1) -> To Workspace30/1
  Fy Subsystem/1(Out1) -> To Workspace31/1
  Fz Subsystem/1(Out1) -> To Workspace9/1
  Omega Subsystem/1(Out1) -> To Workspace7/1
  Bus Selector5/1 -> To Workspace5/1
  Bus Selector6/1 -> To Workspace6/1
  Bus Selector22/1 -> To Workspace1/1
  Bus Selector26/1 -> To Workspace28/1
  Bus Selector25/1 -> To Workspace27/1
  In1/1 -> Bus Selector6/1, Bus Selector1/1, Bus Selector4/1, Bus Selector11/1, Fx Subsystem/1(In1), Bus Selector22/1, Fy Subsystem/1(In1), Fz Subsystem/1(In1), Mz Subsystem/1(In1), Bus Selector20/1, Bus Selector21/1, Bus Selector24/1, Bus Selector23/1, Bus Selector26/1, Bus Selector19/1, Bus Selector14/1, Bus Selector25/1, Bus Selector13/1, Bus Selector18/1, Bus Selector12/1, Bus Selector17/1, Bus Selector10/1, Bus Selector16/1, Bus Selector9/1, Bus Selector15/1, Bus Selector8/1, Omega Subsystem/1(In1), Bus Selector7/1, Bus Selector5/1, Bus Selector2/1, Bus Selector3/1
  Bus Selector8/1 -> To Workspace12/1
  Bus Selector9/1 -> To Workspace13/1
  Bus Selector10/1 -> To Workspace14/1
  Bus Selector12/1 -> To Workspace15/1
  Bus Selector13/1 -> To Workspace16/1
  Bus Selector14/1 -> To Workspace17/1
  Bus Selector15/1 -> To Workspace18/1
  Bus Selector16/1 -> To Workspace19/1
  Bus Selector17/1 -> To Workspace20/1
  Bus Selector18/1 -> To Workspace21/1
  Bus Selector19/1 -> To Workspace22/1
  Mz Subsystem/1(Out1) -> To Workspace23/1
  Bus Selector20/1 -> To Workspace24/1
  Bus Selector21/1 -> To Workspace25/1
  Bus Selector23/1 -> To Workspace26/1
  Bus Selector24/1 -> To Workspace29/1

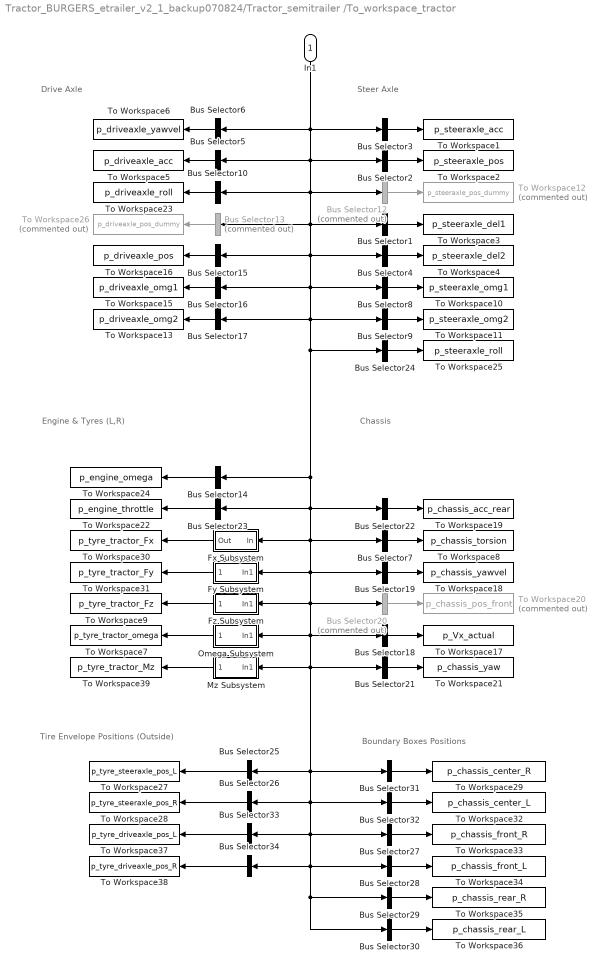
== system Tractor_BURGERS_etrailer_v2_1_backup070824/Tractor_semitrailer /To_workspace_tractor ==
  note: Tire Envelope Positions (Outside)
  note: Engine & Tyres (L,R)
  note: Chassis
  note: Steer Axle
  note: Drive Axle
  note: Boundary Boxes Positions
  In1 : Inport
  Bus Selector1 : BusSelector  OutputSignals=steeraxle.Delta 1_L  OutputAsBus=on
  Bus Selector10 : BusSelector  OutputSignals=driveaxle.roll  OutputAsBus=on
  Bus Selector12 : BusSelector  Commented=on  OutputSignals=steeraxle.Dummyaxle_pos  OutputAsBus=on
  Bus Selector13 : BusSelector  Commented=on  OutputSignals=driveaxle.G2_Driveaxle_pos_dummy  OutputAsBus=on
  Bus Selector14 : BusSelector  OutputSignals=driveline.omega  OutputAsBus=on
  Bus Selector15 : BusSelector  OutputSignals=driveaxle.pos  OutputAsBus=on
  Bus Selector16 : BusSelector  OutputSignals=driveaxle.Omega1  OutputAsBus=on
  Bus Selector17 : BusSelector  OutputSignals=driveaxle.Omega2  OutputAsBus=on
  Bus Selector18 : BusSelector  OutputSignals=chassis.Vx  OutputAsBus=on
  Bus Selector19 : BusSelector  OutputSignals=chassis.yawvel  OutputAsBus=on
  Bus Selector2 : BusSelector  OutputSignals=steeraxle.pos  OutputAsBus=on
  Bus Selector20 : BusSelector  Commented=on  OutputSignals=chassis.pos_chassis frt  OutputAsBus=on
  Bus Selector21 : BusSelector  OutputSignals=chassis.Yaw  OutputAsBus=on
  Bus Selector22 : BusSelector  OutputSignals=chassis.centre_acc  OutputAsBus=on
  Bus Selector23 : BusSelector  OutputSignals=driveline.throttle  OutputAsBus=on
  Bus Selector24 : BusSelector  OutputSignals=steeraxle.roll  OutputAsBus=on
  Bus Selector25 : BusSelector  OutputSignals=steeraxle.T_L_pos.x,steeraxle.T_L_pos.y,steeraxle.T_L_pos.z  OutputAsBus=on
  Bus Selector26 : BusSelector  OutputSignals=steeraxle.T_R_pos.x,steeraxle.T_R_pos.y,steeraxle.T_R_pos.z  OutputAsBus=on
  Bus Selector27 : BusSelector  OutputSignals=chassis.Boundary.pos_FR  OutputAsBus=on
  Bus Selector28 : BusSelector  OutputSignals=chassis.Boundary.pos_FL  OutputAsBus=on
  Bus Selector29 : BusSelector  OutputSignals=chassis.Boundary.pos_RR  OutputAsBus=on
  Bus Selector3 : BusSelector  OutputSignals=steeraxle.acc  OutputAsBus=on
  Bus Selector30 : BusSelector  OutputSignals=chassis.Boundary.pos_RL  OutputAsBus=on
  Bus Selector31 : BusSelector  OutputSignals=chassis.Boundary.pos_CR  OutputAsBus=on
  Bus Selector32 : BusSelector  OutputSignals=chassis.Boundary.pos_CL  OutputAsBus=on
  Bus Selector33 : BusSelector  OutputSignals=driveaxle.T_L1_pos  OutputAsBus=on
  Bus Selector34 : BusSelector  OutputSignals=driveaxle.T_R1_pos  OutputAsBus=on
  Bus Selector4 : BusSelector  OutputSignals=steeraxle.Delta 2_R  OutputAsBus=on
  Bus Selector5 : BusSelector  OutputSignals=driveaxle.acc  OutputAsBus=on
  Bus Selector6 : BusSelector  OutputSignals=chassis.yawvel  OutputAsBus=on
  Bus Selector7 : BusSelector  OutputSignals=chassis.torsion  OutputAsBus=on
  Bus Selector8 : BusSelector  OutputSignals=steeraxle.Omega1  OutputAsBus=on
  Bus Selector9 : BusSelector  OutputSignals=steeraxle.Omega2  OutputAsBus=on
  Fx Subsystem : Subsystem
      mask Display: disp('Fx');
  Fy Subsystem : Subsystem
      mask Display: disp('Fy');
  Fz Subsystem : Subsystem
      mask Display: disp('Fz');
  Mz Subsystem : Subsystem
      mask Display: disp('Mz');
  Omega Subsystem : Subsystem
      mask Display: disp('Ω');
  To Workspace1 : ToWorkspace  VariableName=p_steeraxle_acc  SampleTime=sp_t
  To Workspace10 : ToWorkspace  VariableName=p_steeraxle_omg1  SampleTime=sp_t
  To Workspace11 : ToWorkspace  VariableName=p_steeraxle_omg2  SampleTime=sp_t
  To Workspace12 : ToWorkspace  Commented=on  VariableName=p_steeraxle_pos_dummy  SampleTime=-1
  To Workspace13 : ToWorkspace  VariableName=p_driveaxle_omg2  SampleTime=sp_t
  To Workspace15 : ToWorkspace  VariableName=p_driveaxle_omg1  SampleTime=sp_t
  To Workspace16 : ToWorkspace  VariableName=p_driveaxle_pos  SampleTime=sp_t
  To Workspace17 : ToWorkspace  VariableName=p_Vx_actual  SampleTime=sp_t
  To Workspace18 : ToWorkspace  VariableName=p_chassis_yawvel  SampleTime=sp_t
  To Workspace19 : ToWorkspace  VariableName=p_chassis_acc_rear  SampleTime=sp_t
  To Workspace2 : ToWorkspace  VariableName=p_steeraxle_pos  SampleTime=sp_t
  To Workspace20 : ToWorkspace  Commented=on  VariableName=p_chassis_pos_front  SampleTime=-1
  To Workspace21 : ToWorkspace  VariableName=p_chassis_yaw  SampleTime=sp_t
  To Workspace22 : ToWorkspace  VariableName=p_engine_throttle  SampleTime=sp_t
  To Workspace23 : ToWorkspace  VariableName=p_driveaxle_roll  SampleTime=sp_t
  To Workspace24 : ToWorkspace  VariableName=p_engine_omega  SampleTime=sp_t
  To Workspace25 : ToWorkspace  VariableName=p_steeraxle_roll  SampleTime=sp_t
  To Workspace26 : ToWorkspace  Commented=on  VariableName=p_driveaxle_pos_dummy  SampleTime=-1
  To Workspace27 : ToWorkspace  VariableName=p_tyre_steeraxle_pos_L  SampleTime=sp_t
  To Workspace28 : ToWorkspace  VariableName=p_tyre_steeraxle_pos_R  SampleTime=sp_t
  To Workspace29 : ToWorkspace  VariableName=p_chassis_center_R  SampleTime=sp_t
  To Workspace3 : ToWorkspace  VariableName=p_steeraxle_del1  SampleTime=sp_t
  To Workspace30 : ToWorkspace  VariableName=p_tyre_tractor_Fx  SampleTime=sp_t
  To Workspace31 : ToWorkspace  VariableName=p_tyre_tractor_Fy  SampleTime=sp_t
  To Workspace32 : ToWorkspace  VariableName=p_chassis_center_L  SampleTime=sp_t
  To Workspace33 : ToWorkspace  VariableName=p_chassis_front_R  SampleTime=sp_t
  To Workspace34 : ToWorkspace  VariableName=p_chassis_front_L  SampleTime=sp_t
  To Workspace35 : ToWorkspace  VariableName=p_chassis_rear_R  SampleTime=sp_t
  To Workspace36 : ToWorkspace  VariableName=p_chassis_rear_L  SampleTime=sp_t
  To Workspace37 : ToWorkspace  VariableName=p_tyre_driveaxle_pos_L  SampleTime=sp_t
  To Workspace38 : ToWorkspace  VariableName=p_tyre_driveaxle_pos_R  SampleTime=sp_t
  To Workspace39 : ToWorkspace  VariableName=p_tyre_tractor_Mz  SampleTime=sp_t
  To Workspace4 : ToWorkspace  VariableName=p_steeraxle_del2  SampleTime=sp_t
  To Workspace5 : ToWorkspace  VariableName=p_driveaxle_acc  SampleTime=sp_t
  To Workspace6 : ToWorkspace  VariableName=p_driveaxle_yawvel  SampleTime=sp_t
  To Workspace7 : ToWorkspace  VariableName=p_tyre_tractor_omega  SampleTime=sp_t
  To Workspace8 : ToWorkspace  VariableName=p_chassis_torsion  SampleTime=sp_t
  To Workspace9 : ToWorkspace  VariableName=p_tyre_tractor_Fz  SampleTime=sp_t
  wires:
  Bus Selector14/1 -> To Workspace24/1
  Bus Selector18/1 -> To Workspace17/1
  Bus Selector7/1 -> To Workspace8/1
  Bus Selector2/1 -> To Workspace2/1
  Bus Selector3/1 -> To Workspace1/1
  Fx Subsystem/1(Out) -> To Workspace30/1
  Fy Subsystem/1(Out1) -> To Workspace31/1
  Fz Subsystem/1(Out1) -> To Workspace9/1
  Omega Subsystem/1(Out1) -> To Workspace7/1
  Bus Selector1/1 -> To Workspace3/1
  Bus Selector4/1 -> To Workspace4/1
  Bus Selector5/1 -> To Workspace5/1
  Bus Selector6/1 -> To Workspace6/1
  Bus Selector8/1 -> To Workspace10/1
  Bus Selector9/1 -> To Workspace11/1
  Bus Selector12/1 -> To Workspace12/1
  Bus Selector16/1 -> To Workspace15/1
  Bus Selector17/1 -> To Workspace13/1
  Bus Selector15/1 -> To Workspace16/1
  Bus Selector19/1 -> To Workspace18/1
  Bus Selector22/1 -> To Workspace19/1
  Bus Selector20/1 -> To Workspace20/1
  Bus Selector23/1 -> To Workspace22/1
  Bus Selector10/1 -> To Workspace23/1
  Bus Selector24/1 -> To Workspace25/1
  Bus Selector13/1 -> To Workspace26/1
  Bus Selector21/1 -> To Workspace21/1
  Bus Selector25/1 -> To Workspace27/1
  Bus Selector26/1 -> To Workspace28/1
  Bus Selector32/1 -> To Workspace32/1
  Bus Selector30/1 -> To Workspace36/1
  Bus Selector27/1 -> To Workspace33/1
  Bus Selector28/1 -> To Workspace34/1
  In1/1 -> Bus Selector6/1, Bus Selector24/1, Bus Selector30/1, Bus Selector29/1, Bus Selector28/1, Bus Selector34/1, Bus Selector27/1, Bus Selector33/1, Bus Selector32/1, Bus Selector26/1, Bus Selector31/1, Bus Selector25/1, Bus Selector21/1, Mz Subsystem/1(In1), Bus Selector18/1, Omega Subsystem/1(In1), Bus Selector20/1, Fz Subsystem/1(In1), Bus Selector19/1, Fy Subsystem/1(In1), Bus Selector7/1, Fx Subsystem/1(In), Bus Selector22/1, Bus Selector23/1, Bus Selector14/1, Bus Selector17/1, Bus Selector9/1, Bus Selector16/1, Bus Selector8/1, Bus Selector15/1, Bus Selector4/1, Bus Selector13/1, Bus Selector1/1, Bus Selector10/1, Bus Selector12/1, Bus Selector5/1, Bus Selector2/1, Bus Selector3/1
  Bus Selector29/1 -> To Workspace35/1
  Bus Selector31/1 -> To Workspace29/1
  Bus Selector33/1 -> To Workspace37/1
  Bus Selector34/1 -> To Workspace38/1
  Mz Subsystem/1(Out1) -> To Workspace39/1
